simulink model "LoopShapingTOT"  (R2019b)
settings: Solver=ode45  StartTime=0.0  StopTime=5  RelTol=1e-3  EnableMultiTasking=on
values from neighbouring files (symbols this model uses):
  Go = 1/ bode(G_hf*P*G_L,wc)    [LoopShaping_TP.m]
  m = 0.5    [LCS_freq.m]    (also in LoopShaping_TP.m = 2)
  w_hf = 300    [LoopShaping_TP.m]
  w_p = wc / tan(alpha)    [LoopShaping_TP.m]
  w_z = wc* tan(alpha)    [LoopShaping_TP.m]
settings Model: Creator=Kathleeen  LastModifiedBy=Ivan
settings DataIOCC: LimitDataPoints=on  SaveFormat=Array  ReturnWorkspaceOutputs=off
settings OptimizationCC: LifeSpan=inf
settings DebuggingCC: UnderspecifiedInitializationDetection=Classic  MergeDetectMultiDrivingBlocksExec=none  StateNameClashWarn=warning  SFUnexpectedBacktrackingDiag=warning  SFNoUnconditionalDefaultTransitionDiag=warning  SFExecutionAtInitializationDiag=none  ArithmeticOperatorsInVariantConditions=warning
settings HardwareCC: ProdBitPerPointer=32  ProdBitPerSizeT=32  ProdBitPerPtrDiffT=32  ProdLargestAtomicFloat=None  ProdIntDivRoundTo=Undefined  ProdEndianess=Unspecified  ProdWordSize=32  ProdHWDeviceType=32-bit Generic
settings ModelReferenceCC: PropagateSignalLabelsOutOfModel=off
settings SFSimCC: SimUseLocalCustomCode=off  CustomCodeUndefinedFunction=UseInterfaceOnly
settings RTWCC: RTWUseLocalCustomCode=off
settings CodeAppCC: StateflowObjectComments=on
settings GRTTargetCC: TargetLangStandard=C89/C90 (ANSI)  GeneratePreprocessorConditionals=Disable all
settings ConfigComp: CovMetricSettings=dw  CovHtmlReporting=on  CovSaveCumulativeToWorkspaceVar=on  CovSaveSingleToWorkspaceVar=on  CovExternalEMLEnable=off

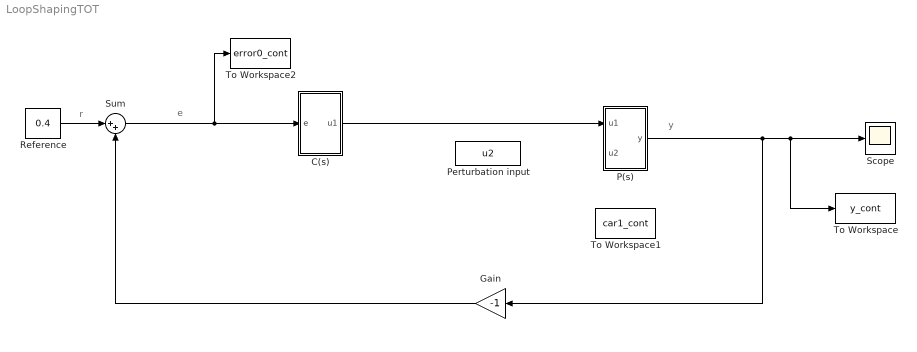
== system LoopShapingTOT ==
  note: e
  note: r
  note: y
  C(s) : Subsystem
  Gain : Gain  Gain=-1
  P(s) : Subsystem
  Perturbation input : FromWorkspace  VariableName=u2  SampleTime=0
  Reference : Constant  Value=0.4
  Scope : Scope
  Sum : Sum  Inputs=|++
  To Workspace : ToWorkspace  VariableName=y_cont  SaveFormat=Timeseries  SampleTime=-1
  To Workspace1 : ToWorkspace  VariableName=car1_cont  SaveFormat=Timeseries  SampleTime=-1
  To Workspace2 : ToWorkspace  VariableName=error0_cont  SaveFormat=Timeseries  SampleTime=-1
  wires:
  Gain/1 -> Sum/2
  Reference/1 -> Sum/1
  Sum/1 -> To Workspace2/1, C(s)/1(e)
  P(s)/1(y) -> Gain/1, To Workspace/1, Scope/1
  C(s)/1(u1) -> P(s)/1(u1)

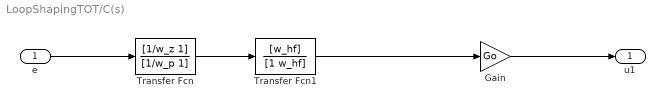
== system LoopShapingTOT/C(s) ==
  e : Inport
  Gain : Gain  Gain=Go
  Transfer Fcn : TransferFcn  Numerator=[1/w_z 1]  Denominator=[1/w_p 1]
  Transfer Fcn1 : TransferFcn  Numerator=[w_hf]  Denominator=[1 w_hf]
  u1 : Outport
  wires:
  e/1 -> Transfer Fcn/1
  Transfer Fcn/1 -> Transfer Fcn1/1
  Gain/1 -> u1/1
  Transfer Fcn1/1 -> Gain/1

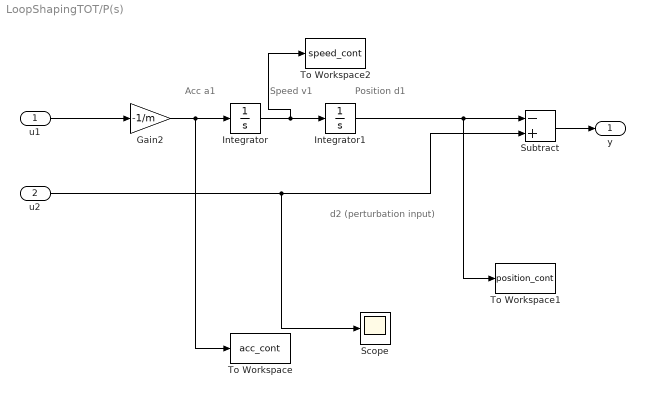
== system LoopShapingTOT/P(s) ==
  note: d2 (perturbation input)
  note: Position d1
  note: Speed v1
  note: Acc a1
  u1 : Inport
  u2 : Inport  Port=2
  Gain2 : Gain  Gain=-1/m
  Integrator : Integrator
  Integrator1 : Integrator
  Scope : Scope
  Subtract : Sum  Inputs=-+
  To Workspace : ToWorkspace  VariableName=acc_cont  SaveFormat=Timeseries  SampleTime=-1
  To Workspace1 : ToWorkspace  VariableName=position_cont  SaveFormat=Timeseries  SampleTime=-1
  To Workspace2 : ToWorkspace  VariableName=speed_cont  SaveFormat=Timeseries  SampleTime=-1
  y : Outport
  wires:
  u1/1 -> Gain2/1
  Subtract/1 -> y/1
  u2/1 -> Scope/1, Subtract/2
  Gain2/1 -> To Workspace/1, Integrator/1
  Integrator/1 -> To Workspace2/1, Integrator1/1
  Integrator1/1 -> To Workspace1/1, Subtract/1
